simulink model "gm_inc_enc_v26_vnl"  (R2022b)
settings: Solver=FixedStepDiscrete  StartTime=0.0  StopTime=SimulationsDauer  RelTol=1e-3
undefined symbols (not defined in the file or in its folder): CW_CCW_Switch, d_axis_hit_CompareValue, DiscIntNeverNeededParam, f_ISR, IncPerTurn, inital_zero_speed_timeout, n_max, Offset_Position_elec, Offset_Position_mech, OmegaPerOverSampl, Periode, Phase_Delay_A, Phase_Delay_B, PolePair, QuadratureFactor, reciprocal_iterations, T_fpga, T_mech
libraries: simulink x25, hdlsllib x11, hdlmdlgenlib x4, dspsrcs4 x3, dspswit3 x2, spsEdgeDetectorLib x2, simulink_extras x1
(part 5 of 5)

== system gm_inc_enc_v26_vnl/IncEnc_V26/speed1/calc_omega_instance4/invt_mult ==
  note: Invert 1/omega and muliply with synchronized oversampling factor
  New_Measurement : Inport  OutDataTypeStr=boolean  PortDimensions=1  SampleTime=1e-08
  rps : Inport  Port=2  OutDataTypeStr=fixdt(1, 38, 32)  PortDimensions=1  SampleTime=1e-08
  Oversampling Factor : Inport  Port=3  OutDataTypeStr=uint16  PortDimensions=1  SampleTime=1e-08
  Data Type Conversion2 : DataTypeConversion  OutDataTypeStr=fixdt(1, 24, 12)  SampleTime=1e-08  SaturateOnIntegerOverflow=off  RndMeth=Floor
  Data Type Conversion3 : DataTypeConversion  OutDataTypeStr=fixdt(0, 6, 0)  SampleTime=1e-08  SaturateOnIntegerOverflow=off  RndMeth=Floor
  Data Type Conversion4 : DataTypeConversion  OutDataTypeStr=fixdt(1, 32, 18)  SampleTime=1e-08  SaturateOnIntegerOverflow=off  RndMeth=Floor
  Div_i1 : Product  Inputs=**  OutDataTypeStr=fixdt(1, 30, 12)  SampleTime=1e-08
  Div_i1_out_dtc : DataTypeConversion  OutDataTypeStr=fixdt(1, 24, 11)  RndMeth=Simplest  SampleTime=1e-08
  HDL Reciprocal : Subsystem
  delayMatch : Delay  DelayLength=double(9)  InitialCondition=0  SampleTime=1e-08
  in_0_pipe : Delay  DelayLength=double(1)  InitialCondition=0  SampleTime=1e-08
  in_1_pipe : Delay  DelayLength=double(1)  InitialCondition=0  SampleTime=1e-08
  out_1_pipe : Delay  DelayLength=double(1)  InitialCondition=0  SampleTime=1e-08
  rd_{0..2,4} (4 alike) : Delay  DelayLength=double(1)  InitialCondition=0  SampleTime=1e-08
  rd_3 : Delay  DelayLength=double(8)  InitialCondition=0  SampleTime=1e-08
  omega_oversampled : Outport  SampleTime=1e-08
  New_Measurement_delayed : Outport  Port=2  SampleTime=1e-08
  wires:
  in_1_pipe/1 -> Data Type Conversion4/1
  out_1_pipe/1 -> delayMatch/1
  in_0_pipe/1 -> out_1_pipe/1
  rd_4/1 -> Div_i1_out_dtc/1
  Div_i1/1 -> rd_4/1
  rd_3/1 -> Div_i1/2
  Data Type Conversion3/1 -> rd_3/1
  Data Type Conversion2/1 -> Div_i1/1
  Div_i1_out_dtc/1 -> rd_2/1
  rd_1/1 -> Data Type Conversion3/1
  rd_0/1 -> Data Type Conversion2/1
  Oversampling Factor/1 -> rd_1/1
  rps/1 -> in_1_pipe/1
  New_Measurement/1 -> in_0_pipe/1
  HDL Reciprocal/1(Out1) -> rd_0/1
  delayMatch/1 -> New_Measurement_delayed/1
  rd_2/1 -> omega_oversampled/1
  Data Type Conversion4/1 -> HDL Reciprocal/1(In1)

== system gm_inc_enc_v26_vnl/IncEnc_V26_vnl/Counter_Theta_el_wOffset/Subsystem/Generate_Increment ==
  Dir_in : Inport
  Constant2 : Constant  OutDataTypeStr=int16  SampleTime=-1
  Constant5 : Constant  Value=-1  OutDataTypeStr=int16  SampleTime=-1
  reset_old1 : Delay  DelayLength=1
  reset_old4 : Delay  DelayLength=1
  speed_old_switch2 : Switch  Threshold=1  SaturateOnIntegerOverflow=off  InputSameDT=off
  Increment : Outport
  wires:
  Constant5/1 -> speed_old_switch2/3
  Constant2/1 -> speed_old_switch2/1
  speed_old_switch2/1 -> reset_old4/1
  reset_old1/1 -> speed_old_switch2/2
  reset_old4/1 -> Increment/1
  Dir_in/1 -> reset_old1/1

== system gm_inc_enc_v26_vnl/IncEnc_V26_vnl/Counter_position_wOffset/Subsystem/Generate_Increment ==
  Dir_in : Inport
  Constant2 : Constant  OutDataTypeStr=int16  SampleTime=-1
  Constant5 : Constant  Value=-1  OutDataTypeStr=int16  SampleTime=-1
  reset_old1 : Delay  DelayLength=1
  reset_old4 : Delay  DelayLength=1
  speed_old_switch2 : Switch  Threshold=1  SaturateOnIntegerOverflow=off  InputSameDT=off
  Increment : Outport
  wires:
  Dir_in/1 -> reset_old1/1
  reset_old4/1 -> Increment/1
  reset_old1/1 -> speed_old_switch2/2
  speed_old_switch2/1 -> reset_old4/1
  Constant2/1 -> speed_old_switch2/1
  Constant5/1 -> speed_old_switch2/3

== system gm_inc_enc_v26_vnl/IncEnc_V26_vnl/speed1/calc_omega/invt_mult ==
  note: Invert 1/omega and muliply with synchronized oversampling factor
  note: At high speed, e.g. at 6000rpm, an steady-state error occurs of around 2.5rpm. I would need more iterrations in the division to get it accurate.
      | However, i also tried to do a multiplication befor the division, so that the Oversampling factor do not gain the steady-state error.
      | But after a try, i still had a steady-state error, which was even bigger (3,2rpm). So i keep it so far.
      | However, the problem is not the fixed-point fromat. The problem is the number of itterations in the division!
      | This applies for 3 iterations
  New_Measurement : Inport
  rps : Inport  Port=2
  Oversampling Factor : Inport  Port=3
  Data Type Conversion1 : DataTypeConversion  Commented=through  OutDataTypeStr=fixdt(1,24,11)  SaturateOnIntegerOverflow=off  RndMeth=Floor
  Data Type Conversion2 : DataTypeConversion  OutDataTypeStr=fixdt(1,24,12)  SaturateOnIntegerOverflow=off  RndMeth=Floor
  Data Type Conversion3 : DataTypeConversion  OutDataTypeStr=fixdt(0,6,0)  SaturateOnIntegerOverflow=off  RndMeth=Floor
  Data Type Conversion4 : DataTypeConversion  OutDataTypeStr=fixdt(1,32,18)  SaturateOnIntegerOverflow=off  RndMeth=Floor
  Div_i1 : Product  Inputs=**  OutDataTypeStr=fixdt(1,24,11)  RndMeth=Simplest  SaturateOnIntegerOverflow=on
  HDL Reciprocal : Reciprocal  NumberOfIterations=reciprocal_iterations
  omega_oversampled : Outport
  New_Measurement_delayed : Outport  Port=2
  wires:
  New_Measurement/1 -> New_Measurement_delayed/1
  Data Type Conversion2/1 -> Div_i1/1  "omega/OS_factor"
  Data Type Conversion3/1 -> Div_i1/2  "before-invert"
  Div_i1/1 -> Data Type Conversion1/1  "omega_oversampled"
  Data Type Conversion1/1 -> omega_oversampled/1
  HDL Reciprocal/1 -> Data Type Conversion2/1  "after-invert"
  Data Type Conversion4/1 -> HDL Reciprocal/1  "before-invert"
  rps/1 -> Data Type Conversion4/1
  Oversampling Factor/1 -> Data Type Conversion3/1

== system gm_inc_enc_v26_vnl/Testfield/Counter_position_wOffset/Subsystem/Generate_Increment ==
  Dir_in : Inport
  Constant2 : Constant  OutDataTypeStr=int16  SampleTime=-1
  Constant5 : Constant  Value=-1  OutDataTypeStr=int16  SampleTime=-1
  reset_old1 : Delay  DelayLength=1
  reset_old4 : Delay  DelayLength=1
  speed_old_switch2 : Switch  Threshold=1  SaturateOnIntegerOverflow=off  InputSameDT=off
  Increment : Outport
  wires:
  Constant5/1 -> speed_old_switch2/3
  Constant2/1 -> speed_old_switch2/1
  speed_old_switch2/1 -> reset_old4/1
  reset_old1/1 -> speed_old_switch2/2
  reset_old4/1 -> Increment/1
  Dir_in/1 -> reset_old1/1

== system gm_inc_enc_v26_vnl/IncEnc_V26/speed1/calc_omega_instance1/invt_mult/HDL Reciprocal ==
  In1 : Inport
  Delay1 : Delay  DelayLength=1
  Delay2 : Delay  DelayLength=6
  HDL Reciprocal : Reciprocal  NumberOfIterations=reciprocal_iterations  SampleTime=1e-08
  Out1 : Outport
  wires:
  In1/1 -> Delay1/1
  Delay1/1 -> HDL Reciprocal/1
  HDL Reciprocal/1 -> Delay2/1
  Delay2/1 -> Out1/1

== system gm_inc_enc_v26_vnl/IncEnc_V26/speed1/calc_omega_instance2/invt_mult/HDL Reciprocal ==
  In1 : Inport
  Delay1 : Delay  DelayLength=1
  Delay2 : Delay  DelayLength=6
  HDL Reciprocal : Reciprocal  NumberOfIterations=reciprocal_iterations  SampleTime=1e-08
  Out1 : Outport
  wires:
  In1/1 -> Delay1/1
  Delay1/1 -> HDL Reciprocal/1
  HDL Reciprocal/1 -> Delay2/1
  Delay2/1 -> Out1/1

== system gm_inc_enc_v26_vnl/IncEnc_V26/speed1/calc_omega_instance3/invt_mult/HDL Reciprocal ==
  In1 : Inport
  Delay1 : Delay  DelayLength=1
  Delay2 : Delay  DelayLength=6
  HDL Reciprocal : Reciprocal  NumberOfIterations=reciprocal_iterations  SampleTime=1e-08
  Out1 : Outport
  wires:
  In1/1 -> Delay1/1
  Delay1/1 -> HDL Reciprocal/1
  HDL Reciprocal/1 -> Delay2/1
  Delay2/1 -> Out1/1

== system gm_inc_enc_v26_vnl/IncEnc_V26/speed1/calc_omega_instance4/invt_mult/HDL Reciprocal ==
  In1 : Inport
  Delay1 : Delay  DelayLength=1
  Delay2 : Delay  DelayLength=6
  HDL Reciprocal : Reciprocal  NumberOfIterations=reciprocal_iterations  SampleTime=1e-08
  Out1 : Outport
  wires:
  Delay2/1 -> Out1/1
  HDL Reciprocal/1 -> Delay2/1
  Delay1/1 -> HDL Reciprocal/1
  In1/1 -> Delay1/1

== matlab function gm_inc_enc_v26_vnl/IncEnc_V26_vnl/speed1/OS_factor_logic/oversample_factor ==
  settings: fimath=fimath('RoundingMethod', 'Floor','OverflowAction', 'Wrap','ProductMode', 'FullPrecision', 'SumMode', 'FullPrecision')
  data: AllowCheckOverSampl input; state_Out output fixdt(0,16,0); ReadBack_Omega input; OverSamplOmega input; state input fixdt(0,16,0); InternalOmega input; InternalOmega_Out output fixdt(1,24,11)
function [state_Out,InternalOmega_Out] = fcn(AllowCheckOverSampl, ReadBack_Omega,OverSamplOmega,state,InternalOmega)

Fq16    = fimath('RoundingMethod', 'Floor', 'OverflowAction', 'Wrap','ProductMode', 'FullPrecision', 'ProductWordLength', 16,'ProductFractionLength', 0,'SumMode','SpecifyPrecision','SumWordLength',16,'SumFractionLength',0);
Fq24    = fimath('RoundingMethod', 'Floor', 'OverflowAction', 'Wrap','ProductMode', 'FullPrecision', 'ProductWordLength', 24,'ProductFractionLength',11,'SumMode','SpecifyPrecision','SumWordLength',24,'SumFractionLength',11);

half    = fi(0.5,false,1,1);

if isempty(InternalOmega)
    InternalOmega = fi(0, 1, 24, 11);
end

%Counter State
if isempty(state)
    state = fi(1, 0, 16, 0);
end

%% Count Up 
% pre-calculate since used in comparison and assignment afterwards
Omega_ADD = fi(add(Fq24,InternalOmega,OverSamplOmega),1,24,11); 
Omega_SUB = fi(sub(Fq24,InternalOmega,OverSamplOmega),1,24,11);

if (ReadBack_Omega > Omega_ADD) && (AllowCheckOverSampl == 1)
    state= fi(add(Fq16,state,fi(1, 0, 16, 0)),0,16,0);   %Count up the measure-state
    InternalOmega = Omega_ADD;
elseif(ReadBack_Omega < Omega_SUB) && (AllowCheckOverSampl == 1)
    state= fi(sub(Fq16,state,fi(1, 0, 16, 0)),0,16,0);   %Count down the measure-state
    InternalOmega = Omega_SUB;
elseif(ReadBack_Omega < (OverSamplOmega*half)) && (AllowCheckOverSampl == 1)
    state = fi(1, 0, 16, 0);
end

%% Output the variables
state_Out = state;
InternalOmega_Out = InternalOmega;

end

== matlab function gm_inc_enc_v26_vnl/IncEnc_V26/speed1/OS_factor_logic/align_oversamples/align_oversamples ==
  settings: fimath=fimath('RoundingMethod', 'Floor','OverflowAction', 'Wrap','ProductMode', 'FullPrecision', 'SumMode', 'FullPrecision')
  data: oversampling_factor input; new_transition input; states input; delay_output output
function delay_output  = fcn(oversampling_factor, new_transition, states)

% Fqint8 = fimath('RoundingMethod', 'Floor', 'OverflowAction', 'Wrap','ProductMode', 'SpecifyPrecision', 'ProductWordLength', 8,'ProductFractionLength',0,'SumMode','SpecifyPrecision','SumWordLength',8,'SumFractionLength',0);
half            = fi(0.5,false,1,1);
three_quarter   = fi(0.75,false,2,2);
persistent delay
if isempty(delay)
    delay    = logical([0 0 0 0]);
end

%% detect current ordering
if(new_transition(1) == 1) % omega_A updated
    
    %% change ordering
    %desired order when dir = +1: A, not B, not A, B => 1, 4, 3, 2
    %desired order when dir = -1: A, B, notA, not B  => 1, 2, 3, 4
    % desired order = omega1=A, omega2, omega3, omega4
    omega2= uint8(4);
    omega3= uint8(3);
    omega4= uint8(2);
    
    zero_logic = logical([0,0,0,0]);
    omega2_reset = zero_logic;
    omega3_reset = zero_logic;
    omega4_reset = zero_logic;
    
    omega2_reset(omega2) = true;
    omega3_reset(omega3) = true;
    omega4_reset(omega4) = true;
    
    omega2_target = uint8(oversampling_factor * half );
    omega3_target = uint8(oversampling_factor * three_quarter);
    omega4_target = uint8(oversampling_factor);
    
    if (oversampling_factor>=2)
        if (all(delay == 0) ) % no delay active
            
            if(states(omega4) ~= omega4_target)
                delay = omega4_reset;
                
            elseif(states(omega3) ~= omega3_target )
                delay = omega3_reset;
                
            elseif(states(omega2) ~= omega2_target )
                delay = omega2_reset;
                
            else
                delay = zero_logic; %final state is reached
            end
            
        else % a delay is already active
            if(         (delay(omega4) == 1 ) && (states(omega4) == (omega4_target-1) ) )
                delay = zero_logic;
            elseif(     (delay(omega3) == 1 ) && (states(omega3) == (omega3_target-1) ) )
                delay = zero_logic;
            %elseif(     isequal(delay, omega2_reset ) && (states(omega2) == (omega2_target-1) ) )
            elseif(     (delay(omega2) == 1 ) && (states(omega2) == (omega2_target-1) ) )
                delay = zero_logic;
            end
        end
    else
        delay = zero_logic;
    end
end

delay_output = delay;

end

== matlab function gm_inc_enc_v26_vnl/IncEnc_V26_vnl/speed1/OS_factor_logic/align_oversamples ==
  settings: fimath=fimath('RoundingMethod', 'Floor','OverflowAction', 'Wrap','ProductMode', 'FullPrecision', 'SumMode', 'FullPrecision')
  data: oversampling_factor input; new_transition input; states input; delay_output output
function delay_output  = fcn(oversampling_factor, new_transition, states)

% Fqint8 = fimath('RoundingMethod', 'Floor', 'OverflowAction', 'Wrap','ProductMode', 'SpecifyPrecision', 'ProductWordLength', 8,'ProductFractionLength',0,'SumMode','SpecifyPrecision','SumWordLength',8,'SumFractionLength',0);
half            = fi(0.5,false,1,1);
three_quarter   = fi(0.75,false,2,2);
persistent delay
if isempty(delay)
    delay    = logical([0 0 0 0]);
end

%% detect current ordering
if(new_transition(1) == 1) % omega_A updated
    
    %% change ordering
    %desired order when dir = +1: A, not B, not A, B => 1, 4, 3, 2
    %desired order when dir = -1: A, B, notA, not B  => 1, 2, 3, 4
    % desired order = omega1=A, omega2, omega3, omega4
    omega2= uint8(4);
    omega3= uint8(3);
    omega4= uint8(2);
    
    zero_logic = logical([0,0,0,0]);
    omega2_reset = zero_logic;
    omega3_reset = zero_logic;
    omega4_reset = zero_logic;
    
    omega2_reset(omega2) = true;
    omega3_reset(omega3) = true;
    omega4_reset(omega4) = true;
    
    omega2_target = uint8(oversampling_factor * half );
    omega3_target = uint8(oversampling_factor * three_quarter);
    omega4_target = uint8(oversampling_factor);
    
    if (oversampling_factor>=2)
        if (all(delay == 0) ) % no delay active
            
            if(states(omega4) ~= omega4_target)
                delay = omega4_reset;
                
            elseif(states(omega3) ~= omega3_target )
                delay = omega3_reset;
                
            elseif(states(omega2) ~= omega2_target )
                delay = omega2_reset;
                
            else
                delay = zero_logic; %final state is reached
            end
            
        else % a delay is already active
            if(         (delay(omega4) == 1 ) && (states(omega4) == (omega4_target-1) ) )
                delay = zero_logic;
            elseif(     (delay(omega3) == 1 ) && (states(omega3) == (omega3_target-1) ) )
                delay = zero_logic;
            %elseif(     isequal(delay, omega2_reset ) && (states(omega2) == (omega2_target-1) ) )
            elseif(     (delay(omega2) == 1 ) && (states(omega2) == (omega2_target-1) ) )
                delay = zero_logic;
            end
        end
    else
        delay = zero_logic;
    end
end

delay_output = delay;

end

== matlab function gm_inc_enc_v26_vnl/IncEnc_V26/speed1/OS_factor_logic/oversample_factor/oversample_factor ==
  settings: fimath=fimath('RoundingMethod', 'Floor','OverflowAction', 'Wrap','ProductMode', 'FullPrecision', 'SumMode', 'FullPrecision')
  data: AllowCheckOverSampl input; state_Out output fixdt(0,16,0); ReadBack_Omega input; OverSamplOmega input; state input fixdt(0,16,0); InternalOmega input; InternalOmega_Out output fixdt(1,24,11)
function [state_Out,InternalOmega_Out] = fcn(AllowCheckOverSampl, ReadBack_Omega,OverSamplOmega,state,InternalOmega)

Fq16    = fimath('RoundingMethod', 'Floor', 'OverflowAction', 'Wrap','ProductMode', 'FullPrecision', 'ProductWordLength', 16,'ProductFractionLength', 0,'SumMode','SpecifyPrecision','SumWordLength',16,'SumFractionLength',0);
Fq24    = fimath('RoundingMethod', 'Floor', 'OverflowAction', 'Wrap','ProductMode', 'FullPrecision', 'ProductWordLength', 24,'ProductFractionLength',11,'SumMode','SpecifyPrecision','SumWordLength',24,'SumFractionLength',11);

half    = fi(0.5,false,1,1);

if isempty(InternalOmega)
    InternalOmega = fi(0, 1, 24, 11);
end

%Counter State
if isempty(state)
    state = fi(1, 0, 16, 0);
end

%% Count Up 
% pre-calculate since used in comparison and assignment afterwards
Omega_ADD = fi(add(Fq24,InternalOmega,OverSamplOmega),1,24,11); 
Omega_SUB = fi(sub(Fq24,InternalOmega,OverSamplOmega),1,24,11);

if (ReadBack_Omega > Omega_ADD) && (AllowCheckOverSampl == 1)
    state= fi(add(Fq16,state,fi(1, 0, 16, 0)),0,16,0);   %Count up the measure-state
    InternalOmega = Omega_ADD;
elseif(ReadBack_Omega < Omega_SUB) && (AllowCheckOverSampl == 1)
    state= fi(sub(Fq16,state,fi(1, 0, 16, 0)),0,16,0);   %Count down the measure-state
    InternalOmega = Omega_SUB;
elseif(ReadBack_Omega < (OverSamplOmega*half)) && (AllowCheckOverSampl == 1)
    state = fi(1, 0, 16, 0);
end

%% Output the variables
state_Out = state;
InternalOmega_Out = InternalOmega;

end
